simulink model "ansimtest"  (Simulink 6.4)
settings: Solver=VariableStepDiscrete  SolverMode=SingleTasking  StartTime=0.0  StopTime=40.0  RelTol=1e-3  AbsTol=1e-6
undefined symbols (not defined in the file or in its folder): ansim
settings Model: LastModifiedBy=changtn
settings DataIOCC: LimitDataPoints=off  Refine=4
settings OptimizationCC: BlockReduction=off  BooleanDataType=off
settings DebuggingCC: SolverPrmCheckMsg=none  StrictBusMsg=None
settings HardwareCC: TargetUnknown=on

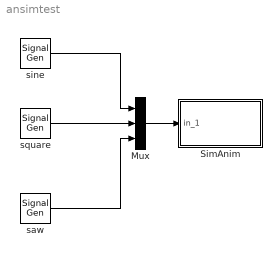
== system ansimtest ==
  Mux : Mux  Inputs=3
  SimAnim : Subsystem
      settings: NameChangeFcn=ansim([],[],[],'NameChange');  OpenFcn=ansimini #Initialize
      mask Type: Simulation Animation
      mask Help: antestdata.mat
      mask Display: disp('Simulation\nAnimation')
  saw : SignalGenerator  WaveForm=sawtooth  Frequency=.4
  sine : SignalGenerator  Frequency=2
  square : SignalGenerator  WaveForm=square  Frequency=.2
  wires:
  Mux/1 -> SimAnim/1(in_1)
  saw/1 -> Mux/3
  sine/1 -> Mux/1
  square/1 -> Mux/2

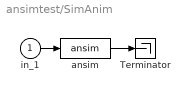
== system ansimtest/SimAnim ==
  in_1 : Inport
  Terminator : Terminator
  ansim : S-Function  LoadFcn=ansim([],[],[],'LoadBlock');  StartFcn=ansim([],[],[],'Start');  StopFcn=ansim([],[],[],'Stop');  FunctionName=ansim  Parameters=1
      settings: CopyFcn=ansim([],[],[],'CopyBlock');  DeleteFcn=ansim([],[],[],'DeleteBlock');
  wires:
  ansim/1 -> Terminator/1
  in_1/1 -> ansim/1
